simulink model "Copy_of_SwingUp"  (R2022b)
settings: Solver=ode1  StartTime=0.0  StopTime=10  FixedStep=0.002  RelTol=1e-3
values from neighbouring files (symbols this model uses):
  g = th(8,1)    [NL_eqns_Disturbance.m]    (also in NL_eqns_EKF.m; StateFcn.m; computeFJacobian.m)
  J_a = th(3,1)    [NL_eqns_Disturbance.m]    (also in NL_eqns_EKF.m; StateFcn.m; computeFJacobian.m)
  K_g = th(9,1)    [NL_eqns_Disturbance.m]    (also in NL_eqns_EKF.m; StateFcn.m; computeFJacobian.m)
  k_m = th(13,1)    [NL_eqns_Disturbance.m]    (also in NL_eqns_EKF.m; StateFcn.m; computeFJacobian.m)
  l_p = th(5,1)    [NL_eqns_Disturbance.m]    (also in NL_eqns_EKF.m; StateFcn.m; computeFJacobian.m)
  m_p = th(6,1)    [NL_eqns_Disturbance.m]    (also in NL_eqns_EKF.m; StateFcn.m; computeFJacobian.m)
  r = th(7,1)    [NL_eqns_Disturbance.m]    (also in NL_eqns_EKF.m; StateFcn.m; computeFJacobian.m)
  Ts = 0.002    [StateFcn.m]
undefined symbols (not defined in the file or in its folder): A_kf, B_kf, c1_tau, C_kf, D_kf, DiscIntNeverNeededParam, E, id_param, Jp_prime, K_lq_en_alpha_eta, K_lq_en_alpha_x, P0, R, voltage_max, x0_down, x0_KF, x0_ob
libraries: simulink x10
settings Model: Creator=federicocorso  LastModifiedBy=federicocorso
settings RTWCC: GenCodeOnly=on

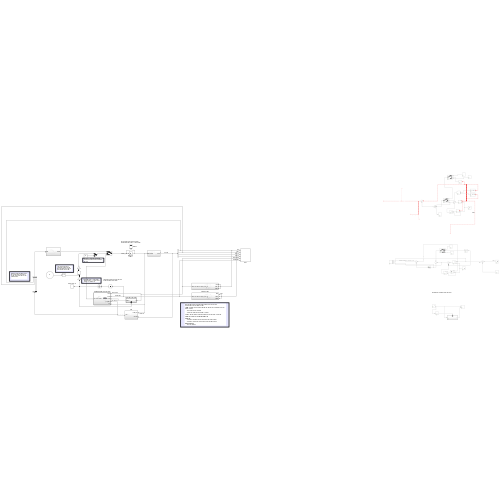
[thumbnail: Simulink's stored preview of the top-level diagram]
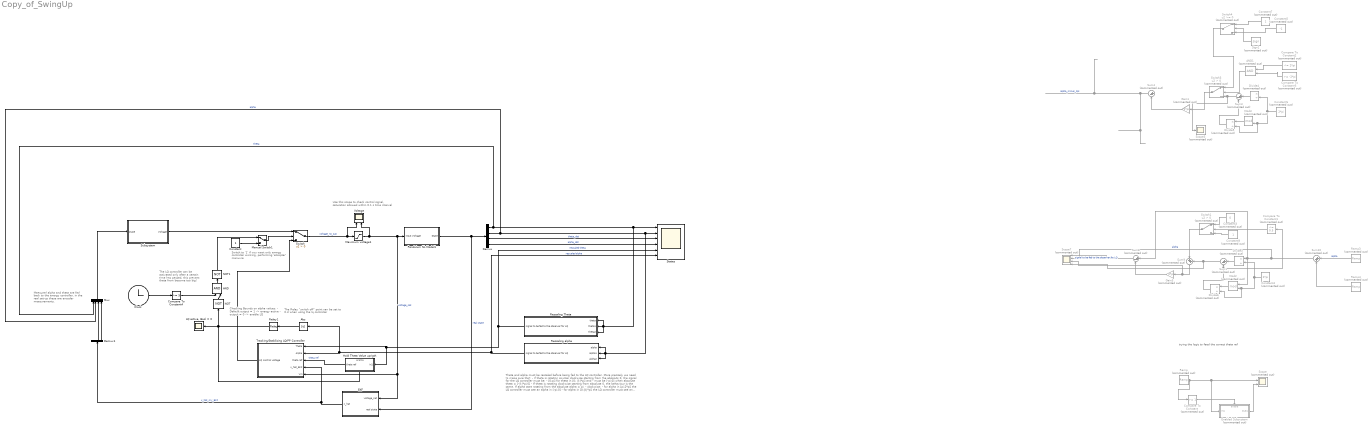
== system Copy_of_SwingUp ==
  note: The Relay "switch off" point can be set to
      | 0.3 when using the lq controller
  note: The LQ controller can be activated only after a certain time has passed, this prevent theta from become too big!
  note: Theta and alpha must be rescaled before being fed to the LQ controller.
      | More precisely we need to make sure that:
      |
      | - if theta is rotating counter clockwise starting from the absolute 0, the signal for the LQ controller must be:
      |
      | - [0;pi] for theta in [0; |k|*pi] and
      |
      | - must be [-pi;0] when absolute theta = [-|k|*pi;0]
      |
      | - If theta is rotating clockwise starting from absolute 0, the behaviour is the same.
      |
      | If alpha start rotating from the absolute alpha = pi:
      |
      | - clockwise:
      | - for alpha in [pi;2*pi] the LQ controller must see an alpha in [-pi;0]
      |
      | - for alpha in [0;|k|*pi] the LQ controller must see an alpha in [0;pi]
      |
      | -counterclockwise:
      | - same as clockwise.
  note: Measured alpha and theta are fed back to the energy controller, in the real set-up these are encoder measurements.
  note: Use this scope to check control signal,
      | saturation allowed within 0.1 s time interval
  note: Switch to '1' if you want only energy
      | controller working, performing 'elicopter'
      | manuvre
  note: Checking Bounds on alpha values:
      | - Default output = 1 -> energy active
      | - output = 0 -> enable LQ
  note: trying the logic to feed the correct theta ref
  AND : Logic  IconShape=distinctive  AllPortsSameDT=off  OutDataTypeStr=boolean
  AND1 : Logic  Commented=on  IconShape=distinctive  AllPortsSameDT=off  OutDataTypeStr=boolean
  Abs : Abs  SaturateOnIntegerOverflow=off
  Clock : Clock
  Compare To Constant : simulink/Logic and Bit Operations/Compare To Constant  Commented=on  relop=>=  const=1  OutDataTypeStr=boolean
  Compare To Constant1 : simulink/Logic and Bit Operations/Compare To Constant  Commented=on  relop=<=  const=0.5  OutDataTypeStr=boolean
  Compare To Constant2 : simulink/Logic and Bit Operations/Compare To Constant  Commented=on  relop=<=  const=2*pi  OutDataTypeStr=boolean
  Compare To Constant3 : simulink/Logic and Bit Operations/Compare To Constant  Commented=on  relop=>=  const=-2*pi  OutDataTypeStr=boolean
  Compare To Constant4 : simulink/Logic and Bit Operations/Compare To Constant  relop=>=  const=5  OutDataTypeStr=boolean
  Constant : Constant
  Constant3 : Constant  Commented=on  Value=0
  Constant4 : Constant  Commented=on  Value=2*pi
  Constant5 : Constant  Commented=on  Value=-1
  Constant6 : Constant  Commented=on  Value=2*pi
  Constant7 : Constant  Commented=on
  Constant9 : Constant  Commented=on
  Demux : Demux
  Demux1 : Demux
  Divide{3..6} (4 alike) : Product  Commented=on  Inputs=*/
  EKF : Subsystem
  Enabled Subsystem : Subsystem  Commented=on  TreatAsAtomicUnit=on
  Gain1 : Gain  Commented=on  Gain=2*pi
  Gain3 : Gain  Commented=on  Gain=2*pi
  Hold Theta Value uprigth : Subsystem  TreatAsAtomicUnit=on
  "LQ active, Bool = 0" : Scope
  Manual Switch1 : ManualSwitch
  Maximum voltage1 : Saturate  UpperLimit=voltage_max  LowerLimit=-voltage_max
  Mod2 : Math  Commented=on  Operator=mod
  Mod3 : Math  Commented=on  Operator=mod
  Mux : Mux
  NOT : Logic  Operator=NOT  IconShape=distinctive  AllPortsSameDT=off  OutDataTypeStr=boolean
  NOT1 : Logic  Operator=NOT  IconShape=distinctive  AllPortsSameDT=off  OutDataTypeStr=boolean
  Pendulum NL Model1 : Subsystem
  Ramp : simulink/Sources/Ramp  Commented=on  slope=1  start=0  InitialOutput=0
  Ramp3 : simulink/Sources/Ramp  Commented=on  slope=pi  start=0  InitialOutput=0
  Ramp4 : simulink/Sources/Ramp  Commented=on  slope=-2*pi  start=3  InitialOutput=0
  Relay1 : Relay  OnSwitchValue=0.5  OffSwitchValue=0.3
  Rescaling Theta : Subsystem
  Rescaling alpha : Subsystem
  Scope : Scope  Commented=on  NumInputPorts=2
  Scope3 : Scope  Commented=on
  Scope7 : Scope  Commented=on  NumInputPorts=4
  Sign1 : Signum  Commented=on
  States : Scope  NumInputPorts=6
  Subsystem : Subsystem
  Sum{1,3..4,8} (4 alike) : Sum  Commented=on  Inputs=|+-
  Sum10 : Sum  Commented=on  Inputs=|++
  Sum9 : Sum  Commented=on  Inputs=|++
  Switch : Switch  Criteria=u2 > Threshold  SaturateOnIntegerOverflow=off  InputSameDT=off
  Switch1 : Switch  Commented=on  Criteria=u2 > Threshold  SaturateOnIntegerOverflow=off  InputSameDT=off
  Switch3 : Switch  Commented=on  Criteria=u2 > Threshold  SaturateOnIntegerOverflow=off  InputSameDT=off
  Switch4 : Switch  Commented=on  SaturateOnIntegerOverflow=off  InputSameDT=off
  Tracking/Stabilizing LQ/PP Controller : Subsystem  TreatAsAtomicUnit=on
  Voltage : Scope  NumInputPorts=2
  wires:
  Demux/1 -> Mux/1, States/1, Rescaling Theta/1(theta), Rescaling Theta/3(theta2), Rescaling Theta/2(theta1)  "theta"
  Pendulum NL Model1/1(State) -> Demux/1, EKF/2(real state)  "real state"
  Switch/1 -> Voltage/1, Maximum voltage1/1  "voltage_no_sat"
  Maximum voltage1/1 -> Pendulum NL Model1/1(Input Voltage), EKF/1(voltage_sat), Tracking/Stabilizing LQ/PP Controller/5(Vm), Voltage/2  "voltage_sat"
  Subsystem/1(Voltage) -> Switch/1
  Demux/2 -> Mux/2, States/2, Rescaling alpha/3(alpha2), Rescaling alpha/2(alpha1), Rescaling alpha/1(alpha)  "alpha"
  Gain1/1 -> Sum4/2
  Sum4/1 -> ?  "alpha_minus_2pi"
  Switch3/1 -> Gain1/1
  Constant5/1 -> Switch4/3
  Divide5/1 -> Sum3/2
  Sign1/1 -> Switch4/2
  Sum3/1 -> Scope3/1, Switch3/3
  Compare To Constant3/1 -> AND1/2
  Divide4/1 -> Sum3/1
  Mod3/1 -> Divide5/1
  Constant6/1 -> Divide5/2, Mod3/2, Divide4/2
  Constant7/1 -> Switch4/1
  ? -> Mod3/1, Divide4/1, Compare To Constant2/1, Sum4/1, Sign1/1, Compare To Constant3/1  "alpha"
  Switch4/1 -> Switch3/1
  Compare To Constant2/1 -> AND1/1
  AND1/1 -> Switch3/2
  Constant3/1 -> Switch1/1
  Divide3/1 -> Sum1/1
  Sum10/1 -> Scope7/2, Sum8/1, Mod2/1, Divide3/1  "alpha"
  Sum1/1 -> Scope7/4, Sum9/2
  Compare To Constant1/1 -> Switch1/2
  Sum8/1 -> Scope7/1  "signal to be fed to the observer for LQ"
  Switch1/1 -> Sum9/1
  Mod2/1 -> Divide6/1
  Ramp3/1 -> Sum10/1  "alpha"
  Sum9/1 -> Scope7/3, Gain3/1
  Constant4/1 -> Divide3/2, Divide6/2, Mod2/2
  Divide6/1 -> Compare To Constant1/1, Sum1/2
  Constant9/1 -> Switch1/3
  Ramp4/1 -> Sum10/2
  Gain3/1 -> Sum8/2
  Tracking/Stabilizing LQ/PP Controller/1(LQ control voltage) -> Switch/3
  Rescaling alpha/1(signal to be fed to the observer for LQ) -> States/6, Tracking/Stabilizing LQ/PP Controller/2(Alpha), Abs/1  "rescaled alpha"
  Rescaling Theta/1(signal to be fed to the observer for LQ) -> States/5, Tracking/Stabilizing LQ/PP Controller/1(Theta), Hold Theta Value uprigth/1(In1)  "rescaled theta"
  Abs/1 -> Relay1/1
  Ramp/1 -> Compare To Constant/1, Enabled Subsystem/1(In1), Scope/1
  Enabled Subsystem/1(Out1) -> Scope/2
  Compare To Constant/1 -> Enabled Subsystem/Enable
  Demux/3 -> States/3  "theta_dot"
  Demux/4 -> States/4  "alpha_dot"
  Hold Theta Value uprigth/1(theta ref) -> Tracking/Stabilizing LQ/PP Controller/3(theta ref)  "theta ref"
  Constant/1 -> Manual Switch1/2
  Demux1/4 -> Mux/4
  Demux1/3 -> Mux/3
  Mux/1 -> Subsystem/1(state)
  Manual Switch1/1 -> Switch/2
  EKF/1(x_hat) -> Tracking/Stabilizing LQ/PP Controller/4(x_hat_EKF), Demux1/1  "x_hat_my_EKF"
  Clock/1 -> Compare To Constant4/1
  Relay1/1 -> NOT/1, "LQ active, Bool = 0"/1, Hold Theta Value uprigth/Enable
  NOT/1 -> AND/2
  Compare To Constant4/1 -> AND/1
  AND/1 -> NOT1/1
  NOT1/1 -> Manual Switch1/1

== system Copy_of_SwingUp/EKF ==
  voltage_sat : Inport
  real state : Inport  Port=2
  Demux1 : Demux
  EKF : Subsystem
  EKF Output : Scope  NumInputPorts=2
  Mux1 : Mux  Inputs=2
  x_hat : Outport
  wires:
  Demux1/2 -> Mux1/2  "alpha"
  Mux1/1 -> EKF/2(y)  "measurements"
  real state/1 -> EKF Output/2, Demux1/1
  Demux1/1 -> Mux1/1  "theta"
  voltage_sat/1 -> EKF/1(V_m)
  EKF/1(x_hat) -> x_hat/1, EKF Output/1  "my_ekf"

== system Copy_of_SwingUp/Enabled Subsystem ==
  In1 : Inport
  Enable : EnablePort
  Out1 : Outport
  wires:
  In1/1 -> Out1/1

== system Copy_of_SwingUp/Hold Theta Value uprigth ==
  In1 : Inport
  Enable : EnablePort
  theta ref : Outport
  wires:
  In1/1 -> theta ref/1

== system Copy_of_SwingUp/Pendulum NL Model1 ==
  note: To perform integration at
      |  discrete time with Eulero Forward
      | substitute this to the integrator block
  Input Voltage : Inport
  Constant : Constant  Value=id_param
  Discrete-Time Integrator1 : DiscreteIntegrator  Commented=on  InitialCondition=x0_down  SampleTime=Ts  ICPrevOutput=DiscIntNeverNeededParam  ICPrevScaledInput=DiscIntNeverNeededParam
  Integrator : Integrator  InitialCondition=x0_down
  MATLAB Function : MATLAB Function  TreatAsAtomicUnit=on
  State : Outport
  wires:
  Input Voltage/1 -> MATLAB Function/2(V_m)
  Constant/1 -> MATLAB Function/3(th)
  MATLAB Function/1(x_dot) -> Integrator/1
  Integrator/1 -> MATLAB Function/1(x), State/1

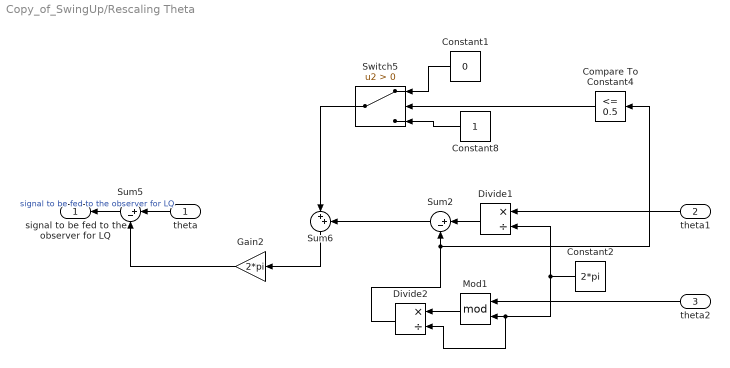
== system Copy_of_SwingUp/Rescaling Theta ==
  theta : Inport
  theta1 : Inport  Port=2
  theta2 : Inport  Port=3
  Compare To Constant4 : simulink/Logic and Bit Operations/Compare To Constant  relop=<=  const=0.5  OutDataTypeStr=boolean
  Constant1 : Constant  Value=0
  Constant2 : Constant  Value=2*pi
  Constant8 : Constant
  Divide1 : Product  Inputs=*/
  Divide2 : Product  Inputs=*/
  Gain2 : Gain  Gain=2*pi
  Mod1 : Math  Operator=mod
  Sum2 : Sum  Inputs=|+-
  Sum5 : Sum  Inputs=|+-
  Sum6 : Sum  Inputs=|++
  Switch5 : Switch  Criteria=u2 > Threshold  SaturateOnIntegerOverflow=off  InputSameDT=off
  signal to be fed to the observer for LQ : Outport
  wires:
  theta/1 -> Sum5/1
  theta1/1 -> Divide1/1
  Divide1/1 -> Sum2/1
  Switch5/1 -> Sum6/1
  Constant8/1 -> Switch5/3
  Divide2/1 -> Compare To Constant4/1, Sum2/2
  Constant1/1 -> Switch5/1
  Mod1/1 -> Divide2/1
  Gain2/1 -> Sum5/2
  Compare To Constant4/1 -> Switch5/2
  Sum5/1 -> signal to be fed to the observer for LQ/1  "signal to be fed to the observer for LQ"
  Sum6/1 -> Gain2/1
  theta2/1 -> Mod1/1
  Constant2/1 -> Divide1/2, Divide2/2, Mod1/2
  Sum2/1 -> Sum6/2

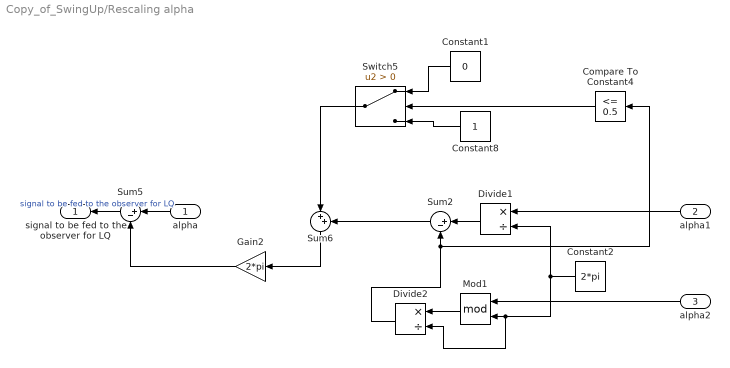
== system Copy_of_SwingUp/Rescaling alpha ==
  alpha : Inport
  alpha1 : Inport  Port=2
  alpha2 : Inport  Port=3
  Compare To Constant4 : simulink/Logic and Bit Operations/Compare To Constant  relop=<=  const=0.5  OutDataTypeStr=boolean
  Constant1 : Constant  Value=0
  Constant2 : Constant  Value=2*pi
  Constant8 : Constant
  Divide1 : Product  Inputs=*/
  Divide2 : Product  Inputs=*/
  Gain2 : Gain  Gain=2*pi
  Mod1 : Math  Operator=mod
  Sum2 : Sum  Inputs=|+-
  Sum5 : Sum  Inputs=|+-
  Sum6 : Sum  Inputs=|++
  Switch5 : Switch  Criteria=u2 > Threshold  SaturateOnIntegerOverflow=off  InputSameDT=off
  signal to be fed to the observer for LQ : Outport
  wires:
  alpha/1 -> Sum5/1
  alpha1/1 -> Divide1/1
  Divide1/1 -> Sum2/1
  Switch5/1 -> Sum6/1
  Constant8/1 -> Switch5/3
  Divide2/1 -> Compare To Constant4/1, Sum2/2
  Constant1/1 -> Switch5/1
  Mod1/1 -> Divide2/1
  Gain2/1 -> Sum5/2
  Compare To Constant4/1 -> Switch5/2
  Sum5/1 -> signal to be fed to the observer for LQ/1  "signal to be fed to the observer for LQ"
  Sum6/1 -> Gain2/1
  alpha2/1 -> Mod1/1
  Constant2/1 -> Divide1/2, Divide2/2, Mod1/2
  Sum2/1 -> Sum6/2

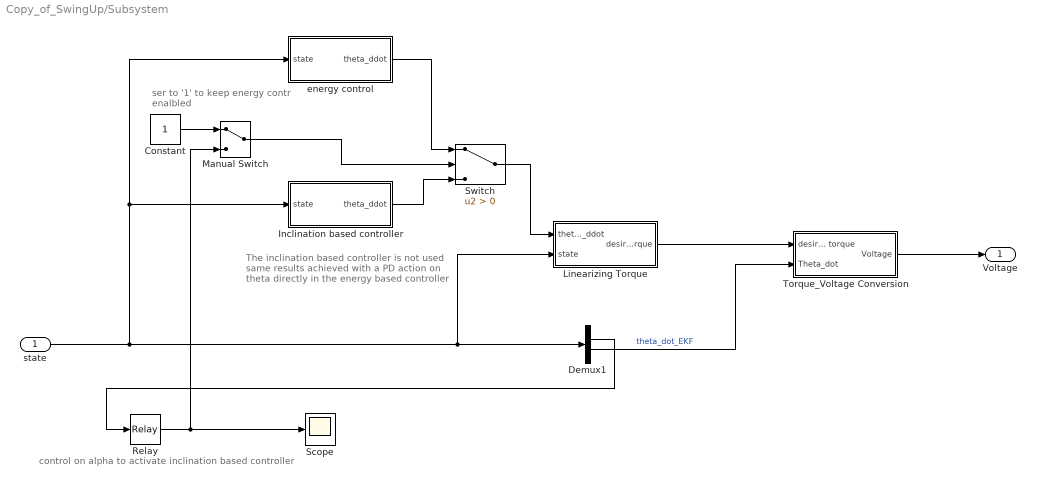
== system Copy_of_SwingUp/Subsystem ==
  note: ser to '1' to keep energy
      | contr enalbled
  note: The inclination based controller is not used
      | same results achieved with a PD action on
      | theta directly in the energy based controller
  note: control on alpha to activate inclination based controller
  state : Inport
  Constant : Constant
  Demux1 : Demux
  Inclination based controller : Subsystem
  Linearizing Torque : Subsystem
  Manual Switch : ManualSwitch
  Relay : Relay  OnSwitchValue=0.6  OffSwitchValue=0.5
  Scope : Scope
  Switch : Switch  Criteria=u2 > Threshold  SaturateOnIntegerOverflow=off  InputSameDT=off
  Torque_Voltage Conversion : Subsystem
  energy control : Subsystem
  Voltage : Outport
  wires:
  Torque_Voltage Conversion/1(Voltage) -> Voltage/1
  Linearizing Torque/1(desired torque) -> Torque_Voltage Conversion/1(desired torque)
  energy control/1(theta_ddot) -> Switch/1
  Demux1/3 -> Torque_Voltage Conversion/2(Theta_dot)  "theta_dot_EKF"
  state/1 -> Linearizing Torque/2(state), Demux1/1, Inclination based controller/1(state), energy control/1(state)
  Switch/1 -> Linearizing Torque/1(theta_ddot)
  Inclination based controller/1(theta_ddot) -> Switch/3
  Constant/1 -> Manual Switch/1
  Manual Switch/1 -> Switch/2
  Relay/1 -> Manual Switch/2, Scope/1
  Demux1/2 -> Relay/1

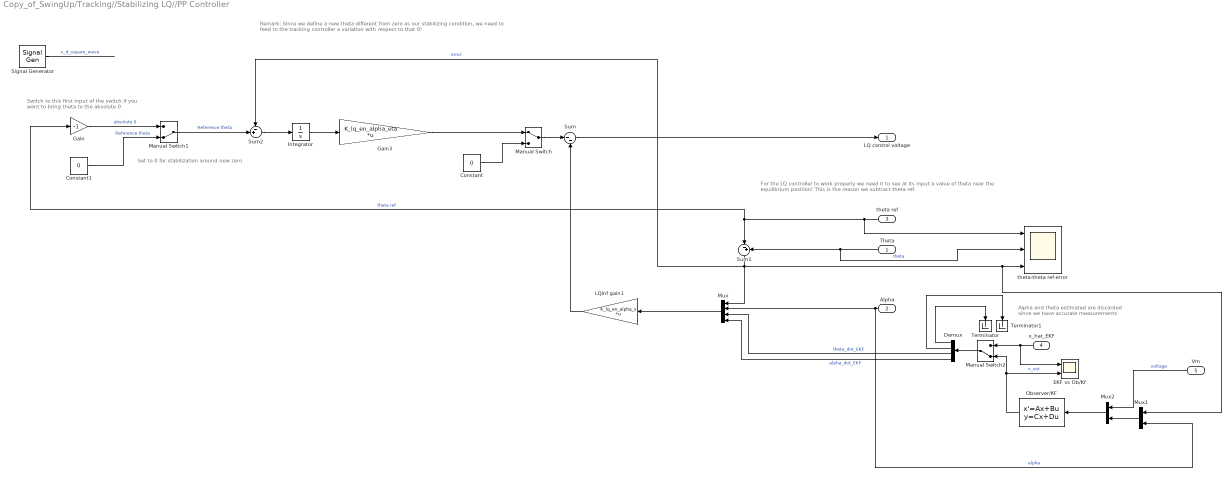
== system Copy_of_SwingUp/Tracking//Stabilizing LQ//PP Controller ==
  note: For the LQ controller to work properly we need it to see at its input a value of theta near the equilibrium position! This is the reason we subtract theta ref.
  note: Switch to this first input of the switch
      | if you want to bring theta to the absolute 0
  note: Remark: Since we define a new theta different from zero as our stabilizing condition, we need to feed to the tracking controller a variation with respect to that 0!
  note: Alpha and theta estimated are discarded
      | since we have accurate measurements
  note: Set to 0 for stabilization around new zero
  Theta : Inport
  Alpha : Inport  Port=2
  theta ref : Inport  Port=3
  x_hat_EKF : Inport  Port=4
  Vm : Inport  Port=5
  Constant : Constant  Value=0
  Constant1 : Constant  Value=0
  Demux : Demux
  EKF vs Ob/Kf : Scope  NumInputPorts=2
  Gain : Gain  Gain=-1
  Gain3 : Gain  Gain=K_lq_en_alpha_eta  Multiplication=Matrix(K*u) (u vector)
  Integrator : Integrator  LimitOutput=on  UpperSaturationLimit=3  LowerSaturationLimit=-3
  LQinf gain1 : Gain  Gain=K_lq_en_alpha_x  Multiplication=Matrix(K*u) (u vector)
  Manual Switch : ManualSwitch
  Manual Switch1 : ManualSwitch  CurrentSetting=0
  Manual Switch2 : ManualSwitch  CurrentSetting=0
  Mux : Mux
  Mux1 : Mux  Inputs=2
  Mux2 : Mux  Inputs=2
  Observer/KF : StateSpace  A=A_kf  B=B_kf  C=C_kf  D=D_kf  InitialCondition=x0_ob
  Signal Generator : SignalGenerator  WaveForm=square  Amplitude=-0.3  Frequency=0.1
  Sum : Sum  Inputs=|--
  Sum1 : Sum  Inputs=|-+
  Sum2 : Sum  Inputs=-+|
  Terminator : Terminator
  Terminator1 : Terminator
  theta-theta ref-error : Scope  NumInputPorts=3
  LQ control voltage : Outport
  wires:
  Mux/1 -> LQinf gain1/1
  LQinf gain1/1 -> Sum/2
  Sum/1 -> LQ control voltage/1
  Demux/1 -> Terminator/1
  Demux/3 -> Mux/3  "theta_dot_EKF"
  Demux/4 -> Mux/4  "alpha_dot_EKF"
  Demux/2 -> Terminator1/1
  theta ref/1 -> Sum1/1, Gain/1, theta-theta ref-error/1  "theta ref"
  Theta/1 -> Sum1/2, theta-theta ref-error/2  "theta"
  Sum1/1 -> Sum2/1, Mux/1, theta-theta ref-error/3, Mux1/1  "error"
  Alpha/1 -> Mux1/2, Mux/2  "alpha"
  Constant/1 -> Manual Switch/2
  Manual Switch/1 -> Sum/1
  Gain3/1 -> Manual Switch/1
  Integrator/1 -> Gain3/1
  Sum2/1 -> Integrator/1
  Constant1/1 -> Manual Switch1/2  "Reference theta"
  Signal Generator/1 -> ?  "x_d_square_wave"
  Manual Switch1/1 -> Sum2/2  "Reference theta"
  Gain/1 -> Manual Switch1/1  "absolute 0"
  Mux2/1 -> Observer/KF/1
  Mux1/1 -> Mux2/2
  Vm/1 -> Mux2/1  "voltage"
  Manual Switch2/1 -> Demux/1
  x_hat_EKF/1 -> Manual Switch2/1, EKF vs Ob/Kf/1
  Observer/KF/1 -> Manual Switch2/2, EKF vs Ob/Kf/2  "x_est"

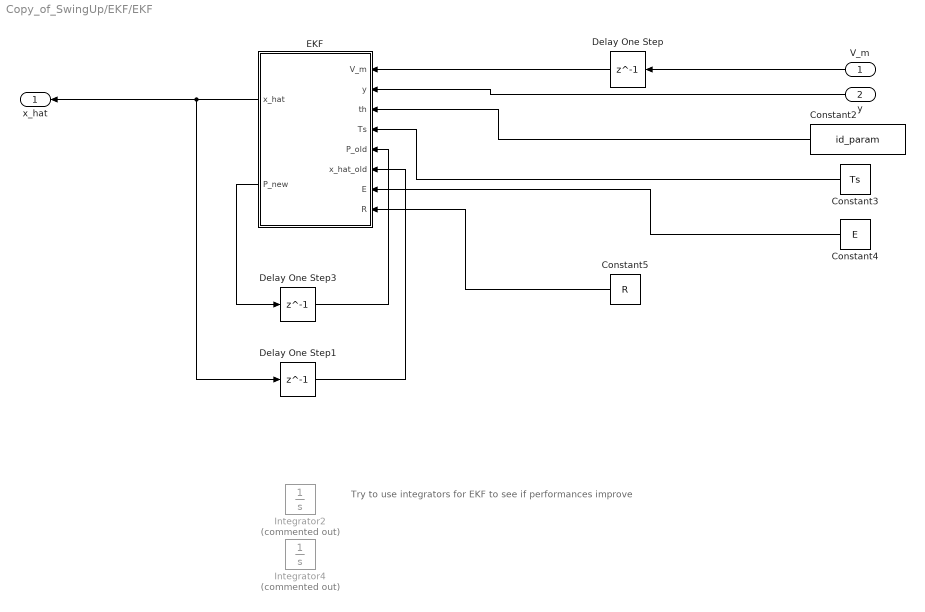
== system Copy_of_SwingUp/EKF/EKF ==
  note: Try to use integrators for EKF to see if performances improve
  V_m : Inport
  y : Inport  Port=2
  Constant2 : Constant  Value=id_param
  Constant3 : Constant  Value=Ts
  Constant4 : Constant  Value=E
  Constant5 : Constant  Value=R
  Delay One Step : Delay  DelayLength=1
  Delay One Step1 : Delay  DelayLength=1  InitialCondition=x0_KF  SampleTime=Ts
  Delay One Step3 : Delay  DelayLength=1  InitialCondition=P0  SampleTime=Ts
  EKF : MATLAB Function  TreatAsAtomicUnit=on
  Integrator2 : Integrator  Commented=on  InitialCondition=P0
  Integrator4 : Integrator  Commented=on  InitialCondition=x0_KF
  x_hat : Outport
  wires:
  Constant5/1 -> EKF/8(R)
  y/1 -> EKF/2(y)
  Constant2/1 -> EKF/3(th)
  EKF/1(x_hat) -> Delay One Step1/1, x_hat/1
  V_m/1 -> Delay One Step/1
  Constant3/1 -> EKF/4(Ts)
  Constant4/1 -> EKF/7(E)
  EKF/2(P_new) -> Delay One Step3/1
  Delay One Step3/1 -> EKF/5(P_old)
  Delay One Step1/1 -> EKF/6(x_hat_old)
  Delay One Step/1 -> EKF/1(V_m)

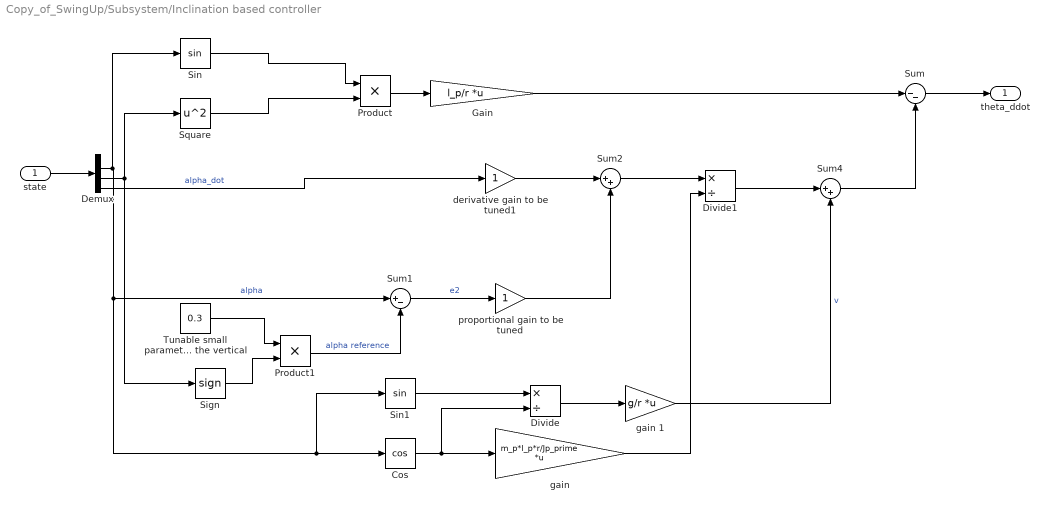
== system Copy_of_SwingUp/Subsystem/Inclination based controller ==
  state : Inport
  Cos : Trigonometry  Operator=cos
  Demux : Demux
  Divide : Product  Inputs=*/
  Divide1 : Product  Inputs=*/
  Gain : Gain  Gain=l_p/r  Multiplication=Matrix(K*u)
  Product : Product
  Product1 : Product
  Sign : Signum
  Sin : Trigonometry
  Sin1 : Trigonometry
  Square : Math  Operator=square
  Sum : Sum  Inputs=|--
  Sum1 : Sum  Inputs=|+-
  Sum2 : Sum  Inputs=|++
  Sum4 : Sum  Inputs=|++
  "Tunable small parameter, angle from the vertical" : Constant  Value=0.3
  derivative gain to be tuned1 : Gain
  "gain " : Gain  Gain=m_p*l_p*r/Jp_prime  Multiplication=Matrix(K*u)
  gain 1 : Gain  Gain=g/r  Multiplication=Matrix(K*u)
  proportional gain to be tuned : Gain
  theta_ddot : Outport
  wires:
  state/1 -> Demux/1
  Sum/1 -> theta_ddot/1
  Gain/1 -> Sum/1
  Product/1 -> Gain/1
  Sin/1 -> Product/1
  Demux/3 -> Sign/1, Square/1
  Square/1 -> Product/2
  Demux/2 -> Sum1/1, Cos/1, Sin1/1, Sin/1  "alpha"
  "Tunable small parameter, angle from the vertical"/1 -> Product1/1
  Sign/1 -> Product1/2
  Product1/1 -> Sum1/2  "alpha reference"
  Sum1/1 -> proportional gain to be tuned/1  "e2"
  Demux/4 -> derivative gain to be tuned1/1  "alpha_dot"
  derivative gain to be tuned1/1 -> Sum2/1
  proportional gain to be tuned/1 -> Sum2/2
  Cos/1 -> "gain "/1, Divide/2
  Sin1/1 -> Divide/1
  Divide/1 -> gain 1/1
  "gain "/1 -> Divide1/2
  gain 1/1 -> Sum4/2  "v"
  Sum2/1 -> Divide1/1
  Divide1/1 -> Sum4/1
  Sum4/1 -> Sum/2

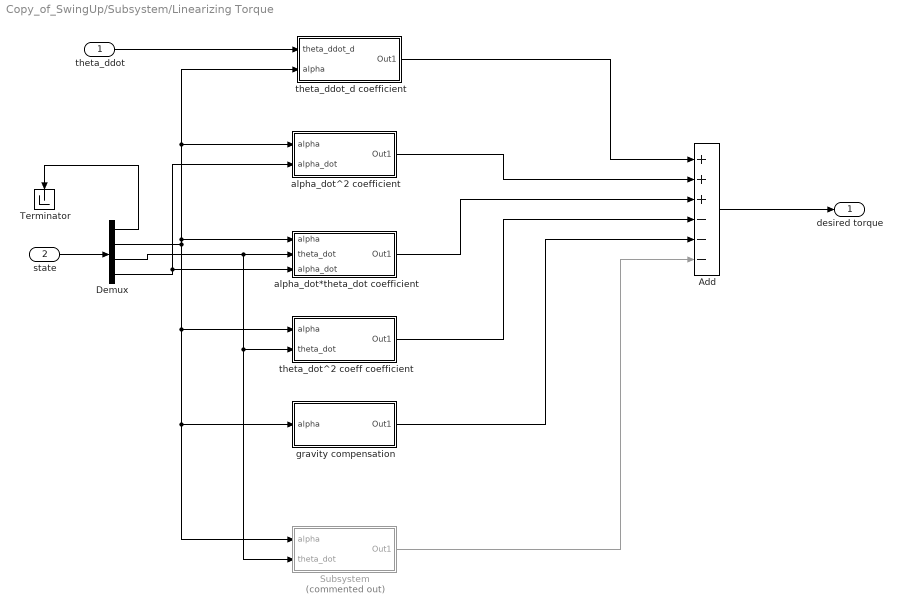
== system Copy_of_SwingUp/Subsystem/Linearizing Torque ==
  theta_ddot : Inport
  state : Inport  Port=2
  Add : Sum  Inputs=+++---
  Demux : Demux
  Subsystem : Subsystem  Commented=on
  Terminator : Terminator
  alpha_dot*theta_dot coefficient : Subsystem
  alpha_dot^2 coefficient : Subsystem
  gravity compensation : Subsystem
  theta_ddot_d coefficient : Subsystem
  theta_dot^2 coeff coefficient : Subsystem
      settings: LibrarySourceBlock=|
      | hdlsllib/Ports &
      | Subsystems/Subsystem
  desired torque : Outport
  wires:
  Add/1 -> desired torque/1
  gravity compensation/1(Out1) -> Add/5
  theta_dot^2 coeff coefficient/1(Out1) -> Add/4
  alpha_dot*theta_dot coefficient/1(Out1) -> Add/3
  alpha_dot^2 coefficient/1(Out1) -> Add/2
  theta_ddot_d coefficient/1(Out1) -> Add/1
  theta_ddot/1 -> theta_ddot_d coefficient/1(theta_ddot_d)
  state/1 -> Demux/1
  Demux/1 -> Terminator/1
  Demux/2 -> Subsystem/1(alpha), gravity compensation/1(alpha), theta_dot^2 coeff coefficient/1(alpha), alpha_dot*theta_dot coefficient/1(alpha), alpha_dot^2 coefficient/1(alpha), theta_ddot_d coefficient/2(alpha)
  Demux/3 -> theta_dot^2 coeff coefficient/2(theta_dot), Subsystem/2(theta_dot), alpha_dot*theta_dot coefficient/2(theta_dot)
  Demux/4 -> alpha_dot*theta_dot coefficient/3(alpha_dot), alpha_dot^2 coefficient/2(alpha_dot)
  Subsystem/1(Out1) -> Add/6

== system Copy_of_SwingUp/Subsystem/Torque_Voltage Conversion ==
  desired torque : Inport
  Theta_dot : Inport  Port=2
  Gain : Gain  Gain=K_g*k_m*c1_tau  Multiplication=Matrix(K*u)
  Sum : Sum  Inputs=|++
  Torque - Voltage proportionality parameter : Gain  Gain=1/c1_tau
  Voltage : Outport
  wires:
  Theta_dot/1 -> Gain/1  "theta dot"
  Torque - Voltage proportionality parameter/1 -> Voltage/1
  Sum/1 -> Torque - Voltage proportionality parameter/1
  Gain/1 -> Sum/2
  desired torque/1 -> Sum/1

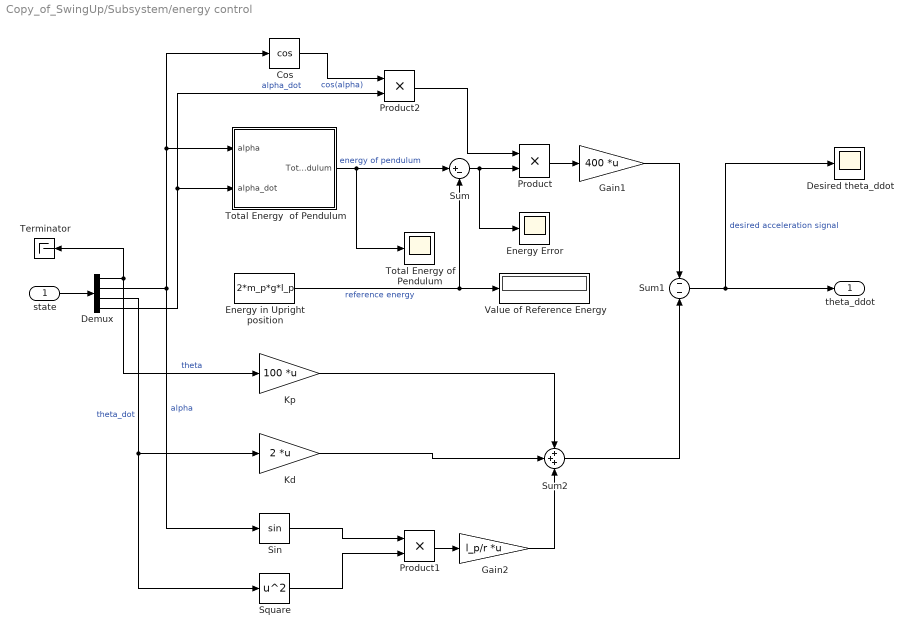
== system Copy_of_SwingUp/Subsystem/energy control ==
  state : Inport
  Cos : Trigonometry  Operator=cos
  Demux : Demux
  Desired theta_ddot : Scope
  Energy Error : Scope
  "Energy in Upright position " : Constant  Value=2*m_p*g*l_p
  Gain1 : Gain  Gain=400  Multiplication=Matrix(K*u)
  Gain2 : Gain  Gain=l_p/r  Multiplication=Matrix(K*u)
  Kd : Gain  Gain=2  Multiplication=Matrix(K*u)
  Kp : Gain  Gain=100  Multiplication=Matrix(K*u)
  Product : Product
  Product1 : Product
  Product2 : Product
  Sin : Trigonometry
  Square : Math  Operator=square
  Sum : Sum  Inputs=|+-
  Sum1 : Sum  Inputs=--
  Sum2 : Sum  Inputs=+++
  Terminator : Terminator
  Total Energy  of Pendulum : Subsystem
  Total Energy of Pendulum : Scope
  Value of Reference Energy : Display
  theta_ddot : Outport
  wires:
  state/1 -> Demux/1
  Demux/2 -> Sin/1, Total Energy  of Pendulum/1(alpha), Cos/1  "alpha"
  Demux/4 -> Total Energy  of Pendulum/2(alpha_dot), Product2/2  "alpha_dot"
  Cos/1 -> Product2/1  "cos(alpha)"
  Product/1 -> Gain1/1
  Gain2/1 -> Sum2/3
  Product1/1 -> Gain2/1
  Demux/3 -> Square/1, Kd/1  "theta_dot"
  Demux/1 -> Kp/1, Terminator/1  "theta"
  Sin/1 -> Product1/1
  Square/1 -> Product1/2
  Total Energy  of Pendulum/1(Total Energy Pendulum) -> Sum/1, Total Energy of Pendulum/1  "energy of pendulum"
  Sum1/1 -> Desired theta_ddot/1, theta_ddot/1  "desired acceleration signal"
  Kp/1 -> Sum2/1
  Kd/1 -> Sum2/2
  Sum2/1 -> Sum1/2
  Gain1/1 -> Sum1/1
  Sum/1 -> Energy Error/1, Product/2
  "Energy in Upright position "/1 -> Value of Reference Energy/1, Sum/2  "reference energy"
  Product2/1 -> Product/1

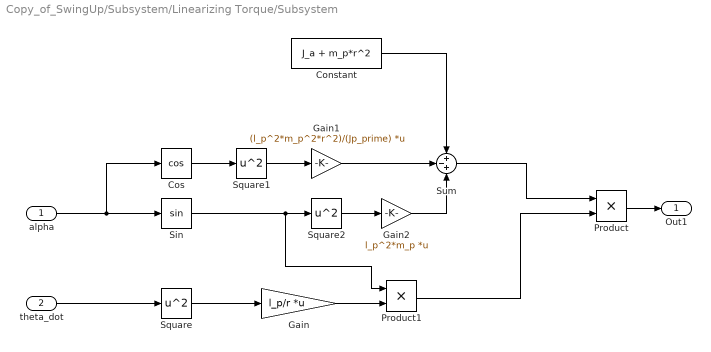
== system Copy_of_SwingUp/Subsystem/Linearizing Torque/Subsystem ==
  alpha : Inport
  theta_dot : Inport  Port=2
  Constant : Constant  Value=J_a + m_p*r^2
  Cos : Trigonometry  Operator=cos
  Gain : Gain  Gain=l_p/r  Multiplication=Matrix(K*u)
  Gain1 : Gain  Gain=(l_p^2*m_p^2*r^2)/(Jp_prime)  Multiplication=Matrix(K*u)
  Gain2 : Gain  Gain=l_p^2*m_p  Multiplication=Matrix(K*u)
  Product : Product
  Product1 : Product
  Sin : Trigonometry
  Square : Math  Operator=square
  Square1 : Math  Operator=square
  Square2 : Math  Operator=square
  Sum : Sum  Inputs=+-+
  Out1 : Outport
  wires:
  theta_dot/1 -> Square/1
  alpha/1 -> Sin/1, Cos/1
  Square/1 -> Gain/1
  Product/1 -> Out1/1
  Gain/1 -> Product1/2
  Sin/1 -> Square2/1, Product1/1
  Cos/1 -> Square1/1
  Square1/1 -> Gain1/1
  Gain1/1 -> Sum/2
  Square2/1 -> Gain2/1
  Gain2/1 -> Sum/3
  Constant/1 -> Sum/1
  Sum/1 -> Product/1
  Product1/1 -> Product/2

== system Copy_of_SwingUp/Subsystem/Linearizing Torque/alpha_dot*theta_dot coefficient ==
  alpha : Inport
  theta_dot : Inport  Port=2
  alpha_dot : Inport  Port=3
  Gain : Gain  Gain=l_p^2*m_p  Multiplication=Matrix(K*u)
  Gain1 : Gain  Gain=2  Multiplication=Matrix(K*u)
  Product : Product
  Product1 : Product
  Sin : Trigonometry
  Out1 : Outport
  wires:
  theta_dot/1 -> Product/1
  alpha_dot/1 -> Product/2
  Gain/1 -> Out1/1
  Product1/1 -> Gain/1
  Product/1 -> Product1/2
  alpha/1 -> Gain1/1
  Gain1/1 -> Sin/1
  Sin/1 -> Product1/1

== system Copy_of_SwingUp/Subsystem/Linearizing Torque/alpha_dot^2 coefficient ==
  alpha : Inport
  alpha_dot : Inport  Port=2
  Gain : Gain  Gain=l_p*m_p*r  Multiplication=Matrix(K*u)
  Product : Product
  Sin : Trigonometry
  Square : Math  Operator=square
  Out1 : Outport
  wires:
  alpha_dot/1 -> Square/1
  Product/1 -> Out1/1
  Square/1 -> Product/2
  alpha/1 -> Sin/1
  Sin/1 -> Gain/1
  Gain/1 -> Product/1

== system Copy_of_SwingUp/Subsystem/Linearizing Torque/gravity compensation ==
  alpha : Inport
  Cos : Trigonometry  Operator=cos
  Gain : Gain  Gain=(g*l_p^2*m_p^2*r)/Jp_prime  Multiplication=Matrix(K*u)
  Product : Product
  Sin : Trigonometry
  Out1 : Outport
  wires:
  Gain/1 -> Out1/1
  Product/1 -> Gain/1
  Cos/1 -> Product/1
  Sin/1 -> Product/2
  alpha/1 -> Cos/1, Sin/1

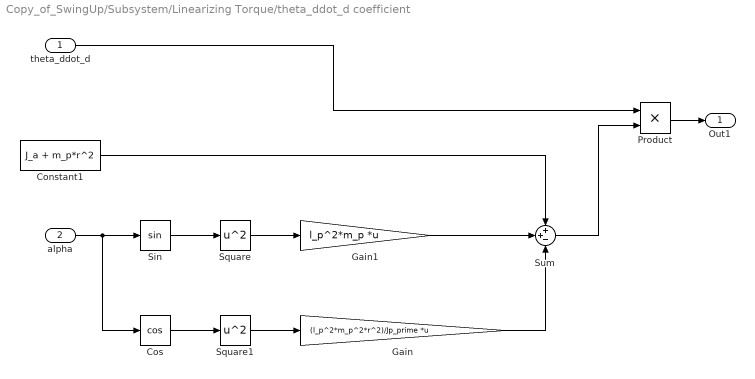
== system Copy_of_SwingUp/Subsystem/Linearizing Torque/theta_ddot_d coefficient ==
  theta_ddot_d : Inport
  alpha : Inport  Port=2
  Constant1 : Constant  Value=J_a + m_p*r^2
  Cos : Trigonometry  Operator=cos
  Gain : Gain  Gain=(l_p^2*m_p^2*r^2)/Jp_prime  Multiplication=Matrix(K*u)
  Gain1 : Gain  Gain=l_p^2*m_p  Multiplication=Matrix(K*u)
  Product : Product
  Sin : Trigonometry
  Square : Math  Operator=square
  Square1 : Math  Operator=square
  Sum : Sum  Inputs=++-
  Out1 : Outport
  wires:
  Product/1 -> Out1/1
  theta_ddot_d/1 -> Product/1
  Sin/1 -> Square/1
  alpha/1 -> Sin/1, Cos/1
  Cos/1 -> Square1/1
  Square/1 -> Gain1/1
  Square1/1 -> Gain/1
  Constant1/1 -> Sum/1
  Gain1/1 -> Sum/2
  Gain/1 -> Sum/3
  Sum/1 -> Product/2

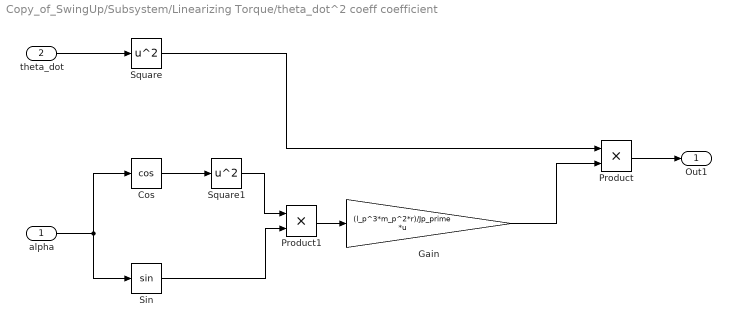
== system Copy_of_SwingUp/Subsystem/Linearizing Torque/theta_dot^2 coeff coefficient ==
  alpha : Inport
  theta_dot : Inport  Port=2
  Cos : Trigonometry  Operator=cos
  Gain : Gain  Gain=(l_p^3*m_p^2*r)/Jp_prime  Multiplication=Matrix(K*u)
  Product : Product
  Product1 : Product
  Sin : Trigonometry
  Square : Math  Operator=square
  Square1 : Math  Operator=square
  Out1 : Outport
  wires:
  theta_dot/1 -> Square/1
  Product/1 -> Out1/1
  Square/1 -> Product/1
  Cos/1 -> Square1/1
  alpha/1 -> Sin/1, Cos/1
  Product1/1 -> Gain/1
  Square1/1 -> Product1/1
  Sin/1 -> Product1/2
  Gain/1 -> Product/2

== system Copy_of_SwingUp/Subsystem/energy control/Total Energy  of Pendulum ==
  alpha : Inport
  alpha_dot : Inport  Port=2
  Constant : Constant
  Cos : Trigonometry  Operator=cos
  Gain : Gain  Gain=g*m_p*l_p  Multiplication=Matrix(K*u)
  Gain1 : Gain  Gain=(1/2)*Jp_prime
  Square : Math  Operator=square
  Sum : Sum  Inputs=|++
  Sum1 : Sum  Inputs=|++
  Total Energy Pendulum : Outport
  wires:
  alpha/1 -> Cos/1
  Cos/1 -> Sum/1
  Constant/1 -> Sum/2
  Sum/1 -> Gain/1
  Sum1/1 -> Total Energy Pendulum/1
  Gain/1 -> Sum1/1
  alpha_dot/1 -> Square/1
  Square/1 -> Gain1/1
  Gain1/1 -> Sum1/2

== matlab function Copy_of_SwingUp/EKF/EKF/EKF ==
  data: V_m input; x_hat output; y input; th input; Ts input; P_old input; x_hat_old input; E input; R input; P_new output
function [x_hat,P_new] = fcn(V_m,y,th,Ts,P_old,x_hat_old,E,R)
% INPUTS
% V_m: input variable, the voltage
% y: measured state
% th: vector of dynamical parameters of the pendulum
% Ts: sampling time for the DT model used in the filter
% P_old: previous state covariance matrix
% x_hat_old: previous state 
% E process covariance matrix
% R measurement covariance matrix

%% Physical params
B_p = th(1,1);
B_r = th(2,1);
J_a = th(3,1);
J_p = th(4,1);
l_p = th(5,1);
m_p = th(6,1);
r = th(7,1);
g = th(8,1);
K_g = th(9,1);
R_m = th(10,1);
eta_g = th(11,1);
eta_m = th(12,1);
k_m = th(13,1);
k_t = th(14,1);

%% computing state derivative of non linear model
tau = eta_g*K_g*eta_m*k_t*(V_m-K_g*k_m*x_hat_old(3,1))/R_m; % motor torque expression-STATIC

t2 = cos(x_hat_old(2,1));
t3 = sin(x_hat_old(2,1));
t4 = l_p.^2;
t5 = l_p.^3;
t7 = m_p.^2;
t8 = r.^2;
t9 = x_hat_old(2,1).*2.0;
t10 = x_hat_old(3,1).^2;
t11 = x_hat_old(4,1).^2;
t12 = J_a.*J_p;
t6 = t4.^2;
t13 = t2.^2;
t14 = sin(t9);
t15 = J_a.*m_p.*t4;
t16 = J_p.*m_p.*t4;
t17 = J_p.*m_p.*t8;
t20 = t4.*t7.*t8;
t18 = t6.*t7;
t19 = t13.*t16;
t24 = t13.*t20;
t21 = t13.*t18;
t22 = -t19;
t25 = -t24;
t23 = -t21;
t26 = t12+t15+t16+t17+t18+t20+t22+t23+t25;
t27 = 1.0./t26;

x_dot = zeros(4,1);

x_dot(1,1) = x_hat_old(3,1);
x_dot(2,1) = x_hat_old(4,1);
x_dot(3,1) = t27.*(J_p.*tau.*-2.0+B_r.*J_p.*x_hat_old(3,1).*2.0-m_p.*t4.*tau.*2.0+t14.*t16.*x_hat_old(3,1).*x_hat_old(4,1).*2.0+t14.*t18.*x_hat_old(3,1).*x_hat_old(4,1).*2.0+B_r.*m_p.*t4.*x_hat_old(3,1).*2.0+r.*t3.*t5.*t7.*t11.*2.0-g.*r.*t2.*t3.*t4.*t7.*2.0-r.*t2.*t5.*t7.*t10.*t14+B_p.*l_p.*m_p.*r.*t2.*x_hat_old(4,1).*2.0+J_p.*l_p.*m_p.*r.*t3.*t11.*2.0).*(-1.0./2.0);
x_dot(4,1) = t27.*(B_p.*J_a.*x_hat_old(4,1).*2.0-t10.*t14.*t15-t10.*t14.*t18-t10.*t14.*t20+t10.*t14.*t21-g.*t3.*t5.*t7.*2.0+t2.*t3.*t11.*t20.*2.0+B_p.*m_p.*t4.*x_hat_old(4,1).*2.0+B_p.*m_p.*t8.*x_hat_old(4,1).*2.0-J_a.*g.*l_p.*m_p.*t3.*2.0-B_p.*m_p.*t4.*t13.*x_hat_old(4,1).*2.0-g.*l_p.*t3.*t7.*t8.*2.0-l_p.*m_p.*r.*t2.*tau.*2.0+g.*t3.*t5.*t7.*t13.*2.0+B_r.*l_p.*m_p.*r.*t2.*x_hat_old(3,1).*2.0+r.*t2.*t5.*t7.*t14.*x_hat_old(3,1).*x_hat_old(4,1).*2.0).*(-1.0./2.0);

%% %{=============== PREDICTION =============}%
x = x_hat_old + Ts*x_dot; % FW Euler simulation one step ahead
%% computing the local jacobian
t2 = cos(x(2));
t3 = sin(x(2));
t4 = K_g.^2;
t5 = l_p.^2;
t6 = l_p.^3;
t8 = m_p.^2;
t9 = r.^2;
t10 = x(2).*2.0;
t11 = x(2).*3.0;
t12 = x(3).^2;
t13 = x(4).^2;
t14 = J_a.*J_p;
t20 = 1.0./R_m;
t7 = t5.^2;
t15 = cos(t10);
t16 = cos(t11);
t17 = t2.^2;
t18 = sin(t10);
t19 = t3.^2;
t21 = m_p.*t5;
t22 = m_p.*t9;
t29 = t5.*t8.*t9;
t23 = J_a.*t21;
t24 = J_p.*t21;
t25 = J_p.*t22;
t26 = t19-1.0;
t27 = t7.*t8;
t32 = J_p+t21+t22;
t34 = t17.*t29;
t28 = t17.*t24;
t30 = t17.*t27;
t35 = -t34;
t31 = -t28;
t33 = -t30;
t36 = t14+t23+t24+t25+t27+t29+t31+t33+t35;
t37 = 1.0./t36;
t38 = t37.^2;
et1 = -(Ts.*l_p.*m_p.*(J_p.*r.*t2.*t13.*4.0-r.*t2.*t12.*t21+r.*t2.*t13.*t21.*4.0-r.*t12.*t16.*t21.*3.0-B_p.*r.*t3.*x(4).*4.0+J_p.*l_p.*t15.*x(3).*x(4).*8.0-g.*l_p.*m_p.*r.*t15.*4.0+m_p.*t6.*t15.*x(3).*x(4).*8.0))./(t14.*4.0+t23.*4.0+t24.*2.0+t25.*4.0+t27.*2.0+t29.*2.0-t15.*t24.*2.0-t15.*t27.*2.0-t15.*t29.*2.0);
et2 = (Ts.*t18.*t21.*t32.*t38.*(B_r.*J_p.*x(3).*2.0+B_r.*t21.*x(3).*2.0+t18.*t24.*x(3).*x(4).*2.0+t18.*t27.*x(3).*x(4).*2.0-g.*r.*t5.*t8.*t18+r.*t3.*t6.*t8.*t13.*2.0+r.*t3.*t6.*t8.*t12.*t26.*2.0+B_p.*l_p.*m_p.*r.*t2.*x(4).*2.0+J_p.*l_p.*m_p.*r.*t3.*t13.*2.0-K_g.*V_m.*eta_g.*eta_m.*k_t.*t20.*t21.*2.0-J_p.*K_g.*V_m.*eta_g.*eta_m.*k_t.*t20.*2.0+J_p.*eta_g.*eta_m.*k_m.*k_t.*t4.*t20.*x(3).*2.0+eta_g.*eta_m.*k_m.*k_t.*t4.*t20.*t21.*x(3).*2.0))./2.0;
et3 = (Ts.*l_p.*m_p.*t20.*(R_m.*g.*t2.*t21.*3.0+R_m.*g.*t2.*t22.*4.0-R_m.*g.*t16.*t21.*3.0+J_a.*R_m.*g.*t2.*4.0-R_m.*m_p.*t6.*t12.*cos(x(2).*4.0).*2.0-B_p.*R_m.*l_p.*t18.*x(4).*4.0+J_a.*R_m.*l_p.*t12.*t15.*4.0+B_r.*R_m.*r.*t3.*x(3).*4.0+R_m.*l_p.*t12.*t15.*t22.*4.0-R_m.*l_p.*t13.*t15.*t22.*4.0+R_m.*m_p.*t6.*t12.*t15.*2.0-R_m.*r.*t2.*t21.*x(3).*x(4).*2.0-R_m.*r.*t16.*t21.*x(3).*x(4).*6.0-K_g.*V_m.*eta_g.*eta_m.*k_t.*r.*t3.*4.0+eta_g.*eta_m.*k_m.*k_t.*r.*t3.*t4.*x(3).*4.0))./(t14.*4.0+t23.*4.0+t24.*2.0+t25.*4.0+t27.*2.0+t29.*2.0-t15.*t24.*2.0-t15.*t27.*2.0-t15.*t29.*2.0);
et4 = Ts.*t18.*t21.*t32.*t38.*(B_p.*J_a.*x(4).*-2.0-B_p.*t21.*x(4).*2.0-B_p.*t22.*x(4).*2.0+t12.*t18.*t23+t12.*t18.*t27+t12.*t18.*t29-t13.*t18.*t29+B_p.*t17.*t21.*x(4).*2.0+g.*t3.*t6.*t8.*2.0-t2.^3.*t3.*t12.*t27.*2.0-g.*t6.*t8.*(t3-t3.^3).*2.0+J_a.*g.*l_p.*m_p.*t3.*2.0+g.*l_p.*t3.*t8.*t9.*2.0-B_r.*l_p.*m_p.*r.*t2.*x(3).*2.0+r.*t3.*t6.*t8.*t26.*x(3).*x(4).*4.0+K_g.*eta_g.*eta_m.*k_t.*l_p.*m_p.*r.*t2.*t20.*(V_m-K_g.*k_m.*x(3)).*2.0).*(-1.0./2.0);
mt1 = [1.0,0.0,0.0,0.0,0.0,1.0,et1+et2,et3+et4,Ts,0.0,Ts.*t37.*(B_r.*t21.*2.0+B_r.*J_p.*2.0+t18.*t24.*x(4).*2.0+t18.*t27.*x(4).*2.0-r.*t2.*t6.*t8.*t18.*x(3).*2.0+J_p.*eta_g.*eta_m.*k_m.*k_t.*t4.*t20.*2.0+eta_g.*eta_m.*k_m.*k_t.*t4.*t20.*t21.*2.0).*(-1.0./2.0)+1.0,Ts.*t37.*(t18.*t23.*x(3).*-2.0-t18.*t27.*x(3).*2.0-t18.*t29.*x(3).*2.0+t18.*t30.*x(3).*2.0+B_r.*l_p.*m_p.*r.*t2.*2.0+r.*t2.*t6.*t8.*t18.*x(4).*2.0+eta_g.*eta_m.*k_m.*k_t.*l_p.*m_p.*r.*t2.*t4.*t20.*2.0).*(-1.0./2.0),0.0,Ts,-Ts.*l_p.*m_p.*t37.*(B_p.*r.*t2+J_p.*l_p.*t18.*x(3)+J_p.*r.*t3.*x(4).*2.0+m_p.*t6.*t18.*x(3)+r.*t3.*t21.*x(4).*2.0)];
mt2 = [Ts.*t37.*(B_p.*t21.*2.0+B_p.*t22.*2.0+B_p.*J_a.*2.0-B_p.*t17.*t21.*2.0+t2.*t3.*t29.*x(4).*4.0+r.*t3.*t6.*t8.*t17.*x(3).*4.0).*(-1.0./2.0)+1.0];
F_eval = reshape([mt1,mt2],4,4);

F_k = F_eval; % jacobian matrix

%% covariance and output
P_temp = F_k*P_old*(F_k') + E; % update covariance matrix
yK = [x(1);x(2)]; % compute output prediction estimate

%% %{========================================}%
%% %{=============== CORRECTION =============}%

H = eye(2,4); % output matrix
I = eye(4);
% innovation
e =  y - yK; % difference between real meas. and predicted output
Ht = H'; % H transposed, compute just once and use 2 times
S = H*P_temp*Ht + R;  % % residual covariance

% near optimal Kalman Gain
K =  (P_temp*Ht)/S;

% updated state estimate
x_hat = x + K*e; % feedback correction
% updated covariance estimate
P_new = (I-K*H)*P_temp;

== matlab function Copy_of_SwingUp/Pendulum NL Model1/MATLAB Function ==
  data: x input; x_dot output; V_m input; th input
function x_dot = NL_eqns(x,V_m,th)
%NL_eqns
%    NL_DIFF_EQNS_SS = NL_eqns(B_p,B_r,J_a,J_p,G,L_P,M_P,R,TAU,x(2,1),x(3,1),x(4,1),X_DOT_1,X_DOT_2,X_DOT_3,X_DOT_4)

%    This function was generated by the Symbolic Math Toolbox version 9.2.
%    09-Mar-2023 15:34:15
B_p = th(1,1);
B_r = th(2,1);
J_a = th(3,1);
J_p = th(4,1);
l_p = th(5,1);
m_p = th(6,1);
r = th(7,1);
g = th(8,1);
K_g = th(9,1);
R_m = th(10,1);
eta_g = th(11,1);
eta_m = th(12,1);
k_m = th(13,1);
k_t = th(14,1);

tau = eta_g*K_g*eta_m*k_t*(V_m-K_g*k_m*x(3,1))/R_m; % motor torque expression-STATIC

t2 = cos(x(2,1));
t3 = sin(x(2,1));
t4 = l_p.^2;
t5 = l_p.^3;
t7 = m_p.^2;
t8 = r.^2;
t9 = x(2,1).*2.0;
t10 = x(3,1).^2;
t11 = x(4,1).^2;
t12 = J_a.*J_p;
t6 = t4.^2;
t13 = t2.^2;
t14 = sin(t9);
t15 = J_a.*m_p.*t4;
t16 = J_p.*m_p.*t4;
t17 = J_p.*m_p.*t8;
t20 = t4.*t7.*t8;
t18 = t6.*t7;
t19 = t13.*t16;
t24 = t13.*t20;
t21 = t13.*t18;
t22 = -t19;
t25 = -t24;
t23 = -t21;
t26 = t12+t15+t16+t17+t18+t20+t22+t23+t25;
t27 = 1.0./t26;

x_dot = zeros(4,1);

x_dot(1,1) = x(3,1);
x_dot(2,1) = x(4,1);
x_dot(3,1) = t27.*(J_p.*tau.*-2.0+B_r.*J_p.*x(3,1).*2.0-m_p.*t4.*tau.*2.0+t14.*t16.*x(3,1).*x(4,1).*2.0+t14.*t18.*x(3,1).*x(4,1).*2.0+B_r.*m_p.*t4.*x(3,1).*2.0+r.*t3.*t5.*t7.*t11.*2.0-g.*r.*t2.*t3.*t4.*t7.*2.0-r.*t2.*t5.*t7.*t10.*t14+B_p.*l_p.*m_p.*r.*t2.*x(4,1).*2.0+J_p.*l_p.*m_p.*r.*t3.*t11.*2.0).*(-1.0./2.0);
x_dot(4,1) = t27.*(B_p.*J_a.*x(4,1).*2.0-t10.*t14.*t15-t10.*t14.*t18-t10.*t14.*t20+t10.*t14.*t21-g.*t3.*t5.*t7.*2.0+t2.*t3.*t11.*t20.*2.0+B_p.*m_p.*t4.*x(4,1).*2.0+B_p.*m_p.*t8.*x(4,1).*2.0-J_a.*g.*l_p.*m_p.*t3.*2.0-B_p.*m_p.*t4.*t13.*x(4,1).*2.0-g.*l_p.*t3.*t7.*t8.*2.0-l_p.*m_p.*r.*t2.*tau.*2.0+g.*t3.*t5.*t7.*t13.*2.0+B_r.*l_p.*m_p.*r.*t2.*x(3,1).*2.0+r.*t2.*t5.*t7.*t14.*x(3,1).*x(4,1).*2.0).*(-1.0./2.0);
